simulink library "ddm"  (R2021b)
settings: Solver=VariableStepAuto  StartTime=0.0  StopTime=10.0  RelTol=1e-3
undefined symbols (not defined in the file): ADDM_FrTMTqDev_X_Nm, ADDM_RrTMTqDev_X_Nm, ENUM_ADASACCSTA_ERROR, ENUM_ADASACCSTA_OFF, ENUM_ADASACCSTA_STANDBY, ENUM_ALLOWMOV_ALLOWREADY, ENUM_APS, ENUM_BRKSTA_ERROR, ENUM_BRKSTA_OFF, ENUM_BRKSTA_ON, ENUM_BRKSW_INVALID, ENUM_BRKSW_OFF, ENUM_BRKSW_ON, ENUM_CHGPREACTERRSTA_OBCPRE, ENUM_DCDCFAULTSTA_ANYFAULTLV1, ENUM_DCDCFAULTSTA_ANYFAULTLV2, ENUM_DRIVETRAIN_AWD, ENUM_DRIVETRAIN_FWD, ENUM_DRIVETRAIN_RWD, ENUM_EDUDRTSTA_NORMAL, ENUM_EPBERROR_FAILED, ENUM_EPBSTA_APPLIED, ENUM_EPBSTA_RELEASED, ENUM_ESCAPSSta_APSUNAVAILABLE, ENUM_GEARACTUALPOSN_INVALID, ENUM_GEARACTUALPOSN_P, ENUM_HVBATTREADYPRE_READY, ENUM_HWRESETSTA_HWRESETING, ENUM_MCUWARN_LV0, ENUM_MCUWARN_LV1, ENUM_MCUWARN_LV2, ENUM_MCUWARN_LV3, ENUM_MCUWARN_NOERROR, ENUM_OBCFAULTSTA_ANYFAULT, ENUM_PAS_R2F2, ENUM_PDFAULT_BATTPDFAIL, ENUM_PDFAULT_DCDCDISABLE, ENUM_PDFAULT_MCUDISABLE, ENUM_PDFAULT_MCUDISCHRG, ENUM_POWERSTA_OFF, ENUM_POWERSTA_ON, ENUM_POWERSTA_READY, ENUM_POWERSTA_STANDBY, ENUM_PRESSINDI_LOW, ENUM_PUFAULT_BATTUPFAIL, ENUM_PUFAULT_DCDCENABLEFAIL, ENUM_PUFAULT_PRECHRGCHKFAIL, ENUM_PUFAULT_SAFETYCHKFAIL, ENUM_PWRSTASW_OFF, ENUM_PWRSTASW_OFFA, ENUM_PWRSTASW_OFFCHVCHRG, ENUM_PWRSTASW_OFFCLVCHRG, ENUM_PWRSTASW_ON, ENUM_PWRSTASW_ONHVCHRG, ENUM_PWRSTASW_READY, ENUM_PWRSTASW_STANDBY, ENUM_RAPSErrWarnSta_NORMAL, ENUM_RAPSErrWarnSta_RAPSERRLV1, ENUM_SHIFTCOMMAND_P, ENUM_SHIFTERERRSTA_PBUTTONFAILURE ... (+471)
libraries: hcu_lib x540, simulink x3
(part 24 of 26)

== system ddm/DDM/DDM/VMC_DDM/BMS Signal Error /BMS Signal Error  ==
  note: Test Pass Criteria
  note: Test Detection Criteria
  note: Diagnostics and Fault Handling
  note: Release Condiction After Decision
  task_time_s : Inport
  VDDM_C3BMS6LCCFS_flg : Inport  Port=2
  VDDM_C3BMS6RCCFS_flg : Inport  Port=3
  VDDM_C3BMS6CSCFS_flg : Inport  Port=4
  No_CAN3_BUS_OFF : Inport  Port=5
  VPMM_PowerSta_enum : Inport  Port=6
  VINP_BMSWarn1_flg : Inport  Port=7
  VINP_BMSWarn2_flg : Inport  Port=8
  VINP_BMSWarn3_flg : Inport  Port=9
  DTC_clear_request : Inport  Port=10
  VINP_BMSWarn4_flg : Inport  Port=11
  VINP_BMSWarn5_flg : Inport  Port=12
  VINP_BMSWarn6_flg : Inport  Port=13
  VINP_BMSWarn7_flg : Inport  Port=14
  VINP_BMSWarn8_flg : Inport  Port=15
  Constant : Constant  Value=ENUM_POWERSTA_OFF
  Constant1 : Constant  Value=ENUM_POWERSTA_OFF
  Constant10 : Constant  Value=ZERO_INT
  Constant12 : Constant  Value=KDDM_BMSSigErrDTC_cnt
  Constant16 : Constant  Value=ENUM_POWERSTA_OFF
  Constant17 : Constant  Value=ENUM_POWERSTA_STANDBY
  Constant18 : Constant  Value=TRUE
  Constant19 : Constant  Value=FALSE
  Constant2 : Constant  Value=FALSE
  Constant3 : Constant  Value=FALSE
  Constant4 : Constant  Value=KDDM_BMSSigErrDetTO_s
  Constant5 : Constant  Value=TRUE
  Constant6 : Constant  Value=KDDM_BMSSigErrPassTO_s
  Constant7 : Constant  Value=KDDM_BMSSigErrDTC_cnt
  Constant8 : Constant  Value=KDDM_VMCDiagnosisOffSW_flg
  Constant9 : Constant  Value=KDDM_BMSSigErrPassTO_s
  DTC_Couter1 : hcu_lib/Basic_Blocks/DTC_Couter
  DTC_Info : hcu_lib/Basic_Blocks/DTC_Info
  Equal : RelationalOperator  Operator=~=  OutDataTypeStr=boolean  RndMeth=Simplest
  Equal1 : RelationalOperator  Operator=~=  OutDataTypeStr=boolean  RndMeth=Simplest
  Equal2 : RelationalOperator  Operator===  OutDataTypeStr=boolean  RndMeth=Simplest
  Equal3 : RelationalOperator  OutDataTypeStr=boolean  RndMeth=Simplest
  Equal4 : RelationalOperator  Operator===  OutDataTypeStr=boolean  RndMeth=Simplest
  Logical Operator1 : Logic  Operator=OR  Inputs=4  AllPortsSameDT=off  OutDataTypeStr=boolean
  Logical Operator10 : Logic  AllPortsSameDT=off  OutDataTypeStr=boolean
  Logical Operator16 : Logic  Operator=OR  Inputs=8  AllPortsSameDT=off  OutDataTypeStr=boolean
  Logical Operator{6,17..18,20..22,24} (7 alike) : Logic  Operator=NOT  AllPortsSameDT=off  OutDataTypeStr=boolean
  Logical Operator2 : Logic  Inputs=5  AllPortsSameDT=off  OutDataTypeStr=boolean
  Logical Operator23 : Logic  Inputs=5  AllPortsSameDT=off  OutDataTypeStr=boolean
  Logical Operator4 : Logic  Operator=OR  Inputs=8  AllPortsSameDT=off  OutDataTypeStr=boolean
  Relational Operator : RelationalOperator  Operator=>  OutDataTypeStr=boolean  RndMeth=Simplest
  Switch{2..3,5..6} (4 alike) : Switch  Criteria=u2 ~= 0
  Terminator : Terminator
  Test Detection Criteria : hcu_lib/Basic_Blocks/Test Detection Criteria
  Timer1 : hcu_lib/Basic_Blocks/Timer
  Unit Delay1 : UnitDelay  SampleTime=-1  HasFrameUpgradeWarning=on
  VDDM_BMSSigErrCFS_flg : Outport
  VDDM_BMSSigErrDetDTC_raw32 : Outport  Port=2
  wires:
  [VDDM_BMSSigErrPass_flg] -> Logical Operator1/1
  Switch6/1 -> [VDDM_BMSSigErrCFSRls_flg]  "VDDM_BMSSigErrCFSRls_flg"
  Equal4/1 -> Logical Operator10/2
  Constant17/1 -> Equal4/2
  DTC_Couter1/2 -> Relational Operator/1  "VDDM_BMSSigErrDTC_cnt"
  Unit Delay1/1 -> Equal2/1
  Logical Operator10/1 -> Logical Operator1/2
  Logical Operator1/1 -> Switch6/2
  Constant16/1 -> Equal2/2
  [VPMM_PowerSta_enum] -> Equal4/1
  Constant18/1 -> Switch6/1
  [VDDM_BMSSigErrCFSRls_flg] -> DTC_Couter1/2
  Constant12/1 -> DTC_Couter1/3
  [DTC_clear_request] -> Logical Operator1/3
  [VDDM_BMSSigErrDet_flg] -> DTC_Couter1/1
  Relational Operator/1 -> Terminator/1  "VDDM_BMSSigErrDFS_flg"
  DTC_Couter1/1 -> [VDDM_BMSSigErrCFS_flg]  "VDDM_BMSSigErrCFS_flg"
  Constant10/1 -> Relational Operator/2
  Constant8/1 -> Logical Operator1/4
  [VPMM_PowerSta_enum] -> Unit Delay1/1
  Constant19/1 -> Switch6/3
  Equal2/1 -> Logical Operator10/1
  Equal3/1 -> [VDDM_BMSSigErrPass_flg]  "VDDM_BMSSigErrPass_flg"
  [task_time_s] -> Timer1/3
  Constant4/1 -> Test Detection Criteria/4
  [VINP_BMSWarn8_flg] -> Logical Operator4/8
  [VINP_BMSWarn7_flg] -> Logical Operator4/7
  [VINP_BMSWarn6_flg] -> Logical Operator4/6
  [VINP_BMSWarn5_flg] -> Logical Operator4/5
  [VINP_BMSWarn8_flg] -> Logical Operator16/8
  [VINP_BMSWarn7_flg] -> Logical Operator16/7
  [VINP_BMSWarn6_flg] -> Logical Operator16/6
  [VINP_BMSWarn5_flg] -> Logical Operator16/5
  [VINP_BMSWarn4_flg] -> Logical Operator16/4
  VINP_BMSWarn8_flg/1 -> [VINP_BMSWarn8_flg]
  VINP_BMSWarn7_flg/1 -> [VINP_BMSWarn7_flg]
  VINP_BMSWarn6_flg/1 -> [VINP_BMSWarn6_flg]
  VINP_BMSWarn5_flg/1 -> [VINP_BMSWarn5_flg]
  VINP_BMSWarn4_flg/1 -> [VINP_BMSWarn4_flg]
  DTC_Info/1 -> VDDM_BMSSigErrDetDTC_raw32/1  "VDDM_BMSSigErrDetDTC_raw32"
  [DTC_clear_request] -> DTC_Info/4
  [VDDM_BMSSigErrCFS_flg] -> DTC_Info/3
  [VDDM_BMSSigErrPass_flg] -> DTC_Info/2
  [VDDM_BMSSigErrDet_flg] -> DTC_Info/1
  Switch5/1 -> Test Detection Criteria/1
  [VDDM_BMSSigErrCFSRls_flg] -> Switch5/2
  Constant3/1 -> Switch5/1
  Constant9/1 -> Timer1/4
  Test Detection Criteria/1 -> [VDDM_BMSSigErrDet_flg]  "VDDM_BMSSigErrDet_flg"
  Constant7/1 -> Test Detection Criteria/3
  [task_time_s] -> Test Detection Criteria/2
  task_time_s/1 -> [task_time_s]  "task_time_s"
  Switch3/1 -> Logical Operator6/1, Timer1/2
  Constant1/1 -> Equal1/2
  [No_CAN3_BUS_OFF] -> Logical Operator23/1
  [VDDM_C3BMS6CSCFS_flg] -> Logical Operator24/1
  Logical Operator21/1 -> Logical Operator23/2
  Logical Operator24/1 -> Logical Operator23/4
  [VDDM_C3BMS6RCCFS_flg] -> Logical Operator22/1
  Equal1/1 -> Logical Operator23/5
  Constant5/1 -> Switch3/3
  Logical Operator23/1 -> Switch3/2
  [VPMM_PowerSta_enum] -> Equal1/1
  Logical Operator4/1 -> Switch3/1
  [VDDM_C3BMS6LCCFS_flg] -> Logical Operator21/1
  Logical Operator22/1 -> Logical Operator23/3
  Logical Operator20/1 -> Logical Operator2/4
  Logical Operator18/1 -> Logical Operator2/3
  Logical Operator17/1 -> Logical Operator2/2
  [VINP_BMSWarn3_flg] -> Logical Operator16/3
  [VINP_BMSWarn2_flg] -> Logical Operator16/2
  [VINP_BMSWarn1_flg] -> Logical Operator16/1
  Logical Operator16/1 -> Switch2/1
  [VDDM_C3BMS6CSCFS_flg] -> Logical Operator20/1
  [VDDM_C3BMS6RCCFS_flg] -> Logical Operator18/1
  [VDDM_C3BMS6LCCFS_flg] -> Logical Operator17/1
  Equal/1 -> Logical Operator2/5
  VINP_BMSWarn1_flg/1 -> [VINP_BMSWarn1_flg]
  No_CAN3_BUS_OFF/1 -> [No_CAN3_BUS_OFF]
  VDDM_C3BMS6CSCFS_flg/1 -> [VDDM_C3BMS6CSCFS_flg]
  VINP_BMSWarn2_flg/1 -> [VINP_BMSWarn2_flg]
  VPMM_PowerSta_enum/1 -> [VPMM_PowerSta_enum]
  VDDM_C3BMS6RCCFS_flg/1 -> [VDDM_C3BMS6RCCFS_flg]
  DTC_clear_request/1 -> [DTC_clear_request]
  VDDM_C3BMS6LCCFS_flg/1 -> [VDDM_C3BMS6LCCFS_flg]
  VINP_BMSWarn3_flg/1 -> [VINP_BMSWarn3_flg]
  Timer1/1 -> Equal3/1
  [VPMM_PowerSta_enum] -> Equal/1
  Constant2/1 -> Switch2/3
  Constant/1 -> Equal/2
  Logical Operator6/1 -> Timer1/1
  Logical Operator2/1 -> Switch2/2
  [No_CAN3_BUS_OFF] -> Logical Operator2/1
  Constant6/1 -> Equal3/2
  [VDDM_BMSSigErrCFS_flg] -> VDDM_BMSSigErrCFS_flg/1
  Switch2/1 -> Switch5/3
  [VINP_BMSWarn1_flg] -> Logical Operator4/1
  [VINP_BMSWarn2_flg] -> Logical Operator4/2
  [VINP_BMSWarn3_flg] -> Logical Operator4/3
  [VINP_BMSWarn4_flg] -> Logical Operator4/4

== system ddm/DDM/DDM/VMC_DDM/CCU Signal Error/CCU Signal Error  ==
  note: Test Pass Criteria
  note: Test Detection Criteria
  note: Release Condiction After Decision
  note: Diagnostics and Fault Handling
  task_time_s : Inport
  VDDM_C3CCU2LCCFS_flg : Inport  Port=2
  VDDM_C3CCU2RCCFS_flg : Inport  Port=3
  VDDM_C3CCU2CSCFS_flg : Inport  Port=4
  No_CAN3_BUS_OFF : Inport  Port=5
  VPMM_PowerSta_enum : Inport  Port=6
  VINP_DCDCFaultSta_enum : Inport  Port=7
  DTC_clear_request : Inport  Port=8
  Constant : Constant  Value=ENUM_POWERSTA_OFF
  Constant1 : Constant  Value=ENUM_POWERSTA_OFF
  Constant10 : Constant  Value=FALSE
  Constant12 : Constant  Value=KDDM_CCUSigErrDTC_cnt
  Constant2 : Constant  Value=FALSE
  Constant21 : Constant  Value=ZERO_INT
  Constant3 : Constant  Value=ENUM_DCDCFAULTSTA_ANYFAULTLV1
  Constant30 : Constant  Value=ENUM_POWERSTA_OFF
  Constant31 : Constant  Value=ENUM_POWERSTA_STANDBY
  Constant32 : Constant  Value=TRUE
  Constant37 : Constant  Value=FALSE
  Constant38 : Constant  Value=KDDM_VMCDiagnosisOffSW_flg
  Constant4 : Constant  Value=KDDM_CCUSigErrDetTO_s
  Constant5 : Constant  Value=TRUE
  Constant6 : Constant  Value=KDDM_CCUSigErrPassTO_s
  Constant7 : Constant  Value=KDDM_CCUSigErrDTC_cnt
  Constant8 : Constant  Value=ENUM_DCDCFAULTSTA_ANYFAULTLV1
  Constant9 : Constant  Value=KDDM_CCUSigErrPassTO_s
  DTC_Couter1 : hcu_lib/Basic_Blocks/DTC_Couter
  DTC_Info : hcu_lib/Basic_Blocks/DTC_Info
  Equal : RelationalOperator  Operator=~=  OutDataTypeStr=boolean  RndMeth=Simplest
  Equal1 : RelationalOperator  Operator=~=  OutDataTypeStr=boolean  RndMeth=Simplest
  Equal17 : RelationalOperator  Operator===  OutDataTypeStr=boolean  RndMeth=Simplest
  Equal18 : RelationalOperator  Operator===  OutDataTypeStr=boolean  RndMeth=Simplest
  Equal2 : RelationalOperator  OutDataTypeStr=boolean  RndMeth=Simplest
  Equal3 : RelationalOperator  OutDataTypeStr=boolean  RndMeth=Simplest
  Equal4 : RelationalOperator  OutDataTypeStr=boolean  RndMeth=Simplest
  Logical Operator10 : Logic  AllPortsSameDT=off  OutDataTypeStr=boolean
  Logical Operator{6,17..18,20..22,24} (7 alike) : Logic  Operator=NOT  AllPortsSameDT=off  OutDataTypeStr=boolean
  Logical Operator2 : Logic  Inputs=5  AllPortsSameDT=off  OutDataTypeStr=boolean
  Logical Operator23 : Logic  Inputs=5  AllPortsSameDT=off  OutDataTypeStr=boolean
  Logical Operator4 : Logic  Operator=OR  Inputs=4  AllPortsSameDT=off  OutDataTypeStr=boolean
  Relational Operator : RelationalOperator  Operator=>  OutDataTypeStr=boolean  RndMeth=Simplest
  Switch{2..3,5..6} (4 alike) : Switch  Criteria=u2 ~= 0
  Terminator : Terminator
  Test Detection Criteria : hcu_lib/Basic_Blocks/Test Detection Criteria
  Timer1 : hcu_lib/Basic_Blocks/Timer
  Unit Delay1 : UnitDelay  SampleTime=-1  HasFrameUpgradeWarning=on
  VDDM_CCUSigErrCFS_flg : Outport
  VDDM_CCUSigErrDetDTC_raw32 : Outport  Port=2
  wires:
  Constant31/1 -> Equal18/2
  Switch6/1 -> [VDDM_CCUSigErrCFSRls_flg]  "VDDM_CCUSigErrCFSRls_flg"
  Constant21/1 -> Relational Operator/2
  Constant30/1 -> Equal17/2
  Equal18/1 -> Logical Operator10/2
  [VDDM_CCUSigErrCFSRls_flg] -> DTC_Couter1/2
  [VDDM_CCUSigErrPass_flg] -> Logical Operator4/1
  Logical Operator10/1 -> Logical Operator4/2
  DTC_Couter1/2 -> Relational Operator/1  "VDDM_CCUSigErrDTC_cnt"
  [DTC_clear_request] -> Logical Operator4/3
  Constant32/1 -> Switch6/1
  Constant38/1 -> Logical Operator4/4
  [VPMM_PowerSta_enum] -> Unit Delay1/1
  Unit Delay1/1 -> Equal17/1
  [VPMM_PowerSta_enum] -> Equal18/1
  Logical Operator4/1 -> Switch6/2
  Constant37/1 -> Switch6/3
  Equal17/1 -> Logical Operator10/1
  DTC_Couter1/1 -> [VDDM_CCUSigErrCFS_flg]  "VDDM_CCUSigErrCFS_flg"
  Constant12/1 -> DTC_Couter1/3
  [VDDM_CCUSigErrDet_flg] -> DTC_Couter1/1
  Relational Operator/1 -> Terminator/1  "VDDM_CCUSigErrDFS_flg"
  DTC_Info/1 -> VDDM_CCUSigErrDetDTC_raw32/1  "VDDM_CCUSigErrDetDTC_raw32"
  [DTC_clear_request] -> DTC_Info/4
  [VDDM_CCUSigErrCFS_flg] -> DTC_Info/3
  [VDDM_CCUSigErrPass_flg] -> DTC_Info/2
  [VDDM_CCUSigErrDet_flg] -> DTC_Info/1
  Switch5/1 -> Test Detection Criteria/1
  Constant10/1 -> Switch5/1
  [VDDM_CCUSigErrCFSRls_flg] -> Switch5/2
  Equal4/1 -> Switch3/1
  Constant8/1 -> Equal4/2
  [VINP_DCDCFaultSta_enum] -> Equal4/1
  Equal2/1 -> Switch2/1
  Constant3/1 -> Equal2/2
  Constant9/1 -> Timer1/4
  [task_time_s] -> Timer1/3
  Test Detection Criteria/1 -> [VDDM_CCUSigErrDet_flg]  "VDDM_CCUSigErrDet_flg"
  Constant7/1 -> Test Detection Criteria/3
  Constant4/1 -> Test Detection Criteria/4
  [task_time_s] -> Test Detection Criteria/2
  task_time_s/1 -> [task_time_s]  "task_time_s"
  Switch3/1 -> Logical Operator6/1, Timer1/2
  Constant1/1 -> Equal1/2
  [No_CAN3_BUS_OFF] -> Logical Operator23/1
  [VDDM_C3CCU2CSCFS_flg] -> Logical Operator24/1
  Logical Operator21/1 -> Logical Operator23/2
  Logical Operator24/1 -> Logical Operator23/4
  [VDDM_C3CCU2RCCFS_flg] -> Logical Operator22/1
  Equal1/1 -> Logical Operator23/5
  Constant5/1 -> Switch3/3
  Logical Operator23/1 -> Switch3/2
  [VPMM_PowerSta_enum] -> Equal1/1
  [VDDM_C3CCU2LCCFS_flg] -> Logical Operator21/1
  Logical Operator22/1 -> Logical Operator23/3
  Logical Operator20/1 -> Logical Operator2/4
  Logical Operator18/1 -> Logical Operator2/3
  Logical Operator17/1 -> Logical Operator2/2
  [VINP_DCDCFaultSta_enum] -> Equal2/1
  [VDDM_C3CCU2CSCFS_flg] -> Logical Operator20/1
  [VDDM_C3CCU2RCCFS_flg] -> Logical Operator18/1
  [VDDM_C3CCU2LCCFS_flg] -> Logical Operator17/1
  Equal/1 -> Logical Operator2/5
  VINP_DCDCFaultSta_enum/1 -> [VINP_DCDCFaultSta_enum]
  No_CAN3_BUS_OFF/1 -> [No_CAN3_BUS_OFF]
  VDDM_C3CCU2CSCFS_flg/1 -> [VDDM_C3CCU2CSCFS_flg]
  VPMM_PowerSta_enum/1 -> [VPMM_PowerSta_enum]
  VDDM_C3CCU2RCCFS_flg/1 -> [VDDM_C3CCU2RCCFS_flg]
  DTC_clear_request/1 -> [DTC_clear_request]
  VDDM_C3CCU2LCCFS_flg/1 -> [VDDM_C3CCU2LCCFS_flg]
  Timer1/1 -> Equal3/1
  [VPMM_PowerSta_enum] -> Equal/1
  Constant2/1 -> Switch2/3
  Constant/1 -> Equal/2
  Logical Operator6/1 -> Timer1/1
  Logical Operator2/1 -> Switch2/2
  [No_CAN3_BUS_OFF] -> Logical Operator2/1
  Constant6/1 -> Equal3/2
  [VDDM_CCUSigErrCFS_flg] -> VDDM_CCUSigErrCFS_flg/1
  Equal3/1 -> [VDDM_CCUSigErrPass_flg]  "VDDM_CCUSigErrPass_flg"
  Switch2/1 -> Switch5/3

== system ddm/DDM/DDM/VMC_DDM/ESC Signal Error/ESC Signal Error  ==
  note: Test Detection Criteria
  note: Test Pass Criteria
  note: Release Condiction After Decision
  note: Diagnostics and Fault Handling
  task_time_s : Inport
  No_CAN1_BUS_OFF : Inport  Port=2
  VPMM_PowerSta_enum : Inport  Port=3
  DTC_clear_request : Inport  Port=4
  VINP_ABSFailed_flg : Inport  Port=5
  VINP_TCSFailed_flg : Inport  Port=6
  VINP_ESCFailed_flg : Inport  Port=7
  VINP_HSAFailed_flg : Inport  Port=8
  VINP_AVHFailed_flg : Inport  Port=9
  VINP_MCPressureV_flg : Inport  Port=10
  VINP_BrkSwV_flg : Inport  Port=11
  VINP_BrkPedalPosSta_flg : Inport  Port=12
  VINP_LongAccelV_flg : Inport  Port=13
  VINP_LatAccelV_flg : Inport  Port=14
  VINP_YawRateV_flg : Inport  Port=15
  VINP_LRRawWhlSpeedV_flg : Inport  Port=16
  VINP_RRRawWhlSpeedV_flg : Inport  Port=17
  VINP_LFRawWhlSpeedV_flg : Inport  Port=18
  VINP_RFRawWhlSpeedV_flg : Inport  Port=19
  VINP_VehSpeed_kph : Inport  Port=20
  VINP_FrntAxlTrqReqDrv_Nm : Inport  Port=21
  VINP_RearAxlTrqReqDrv_Nm : Inport  Port=22
  VDDM_ESC1Err_flg : Inport  Port=23
  VDDM_ESC5Err_flg : Inport  Port=24
  VINP_GRADE_Deg : Inport  Port=25
  VINP_FrntAxlTrqReqBrk_Nm : Inport  Port=26
  VINP_RearAxlTrqReqBrk_Nm : Inport  Port=27
  VINP_ESCAPSSta_enum : Inport  Port=28
  AND : Logic  AllPortsSameDT=off  OutDataTypeStr=boolean
  AND1 : Logic  AllPortsSameDT=off  OutDataTypeStr=boolean
  Constant : Constant  Value=ENUM_POWERSTA_OFF
  Constant1 : Constant  Value=ENUM_POWERSTA_OFF
  Constant10 : Constant  Value=ZERO_INT
  Constant11 : Constant  Value=KDDM_VMCDiagnosisOffSW_flg
  Constant12 : Constant  Value=ENUM_POWERSTA_OFF
  Constant13 : Constant  Value=ENUM_POWERSTA_STANDBY
  Constant14 : Constant  Value=TRUE
  Constant15 : Constant  Value=FALSE
  Constant16 : Constant  Value=FALSE
  Constant17 : Constant  Value=45  OutDataTypeStr=single
  Constant18 : Constant  Value=ZERO_FLOAT  OutDataTypeStr=single
  Constant19 : Constant  Value=ZERO_FLOAT  OutDataTypeStr=single
  Constant2 : Constant  Value=FALSE
  Constant20 : Constant  Value=TRUE
  Constant21 : Constant  Value=ENUM_ESCAPSSta_APSUNAVAILABLE  OutDataTypeStr=single
  Constant34 : Constant  Value=KDDM_ESCSigErrDTC_cnt
  Constant4 : Constant  Value=KDDM_ESCSigErrDetTO_s
  Constant5 : Constant  Value=5300  OutDataTypeStr=single
  Constant6 : Constant  Value=KDDM_ESCSigErrPassTO_s
  Constant66 : Constant  Value=255  OutDataTypeStr=single
  Constant7 : Constant  Value=KDDM_ESCSigErrDTC_cnt
  Constant8 : Constant  Value=5300  OutDataTypeStr=single
  Constant9 : Constant  Value=KDDM_ESCSigErrPassTO_s
  DTC_Couter : hcu_lib/Basic_Blocks/DTC_Couter
  DTC_Info : hcu_lib/Basic_Blocks/DTC_Info
  Data Type Conversion{,1..3} (4 alike) : DataTypeConversion  OutDataTypeStr=single
  Equal : RelationalOperator  Operator=~=  OutDataTypeStr=boolean  RndMeth=Simplest
  Equal1 : RelationalOperator  Operator=~=  OutDataTypeStr=boolean  RndMeth=Simplest
  Equal{2,4..5,54} (4 alike) : RelationalOperator  Operator=>  OutDataTypeStr=boolean  RndMeth=Simplest
  Equal3 : RelationalOperator  OutDataTypeStr=boolean  RndMeth=Simplest
  Equal6 : RelationalOperator  Operator===  OutDataTypeStr=boolean  RndMeth=Simplest
  Equal7 : RelationalOperator  Operator===  OutDataTypeStr=boolean  RndMeth=Simplest
  Logical Operator1 : Logic  AllPortsSameDT=off  OutDataTypeStr=boolean
  Logical Operator2 : Logic  AllPortsSameDT=off  OutDataTypeStr=boolean
  Logical Operator6 : Logic  Operator=NOT  AllPortsSameDT=off  OutDataTypeStr=boolean
  Logical Operator8 : Logic  Operator=OR  Inputs=4  AllPortsSameDT=off  OutDataTypeStr=boolean
  Logical Operator9 : Logic  AllPortsSameDT=off  OutDataTypeStr=boolean
  NOT1 : Logic  Operator=NOT  AllPortsSameDT=off  OutDataTypeStr=boolean
  NOT2 : Logic  Operator=NOT  AllPortsSameDT=off  OutDataTypeStr=boolean
  NOT9 : Logic  Operator=NOT  AllPortsSameDT=off  OutDataTypeStr=boolean
  OR : Logic  Operator=OR  Inputs=13  AllPortsSameDT=off  OutDataTypeStr=boolean
  OR1 : Logic  Operator=OR  Inputs=9  AllPortsSameDT=off  OutDataTypeStr=boolean
  OR2 : Logic  Operator=OR  AllPortsSameDT=off  OutDataTypeStr=boolean
  OR3 : Logic  Operator=OR  AllPortsSameDT=off  OutDataTypeStr=boolean
  Relational Operator : RelationalOperator  Operator=>  OutDataTypeStr=boolean  RndMeth=Simplest
  Relational Operator1 : RelationalOperator  Operator=>  OutDataTypeStr=boolean  RndMeth=Simplest
  Relational Operator2 : RelationalOperator  Operator=>  OutDataTypeStr=boolean  RndMeth=Simplest
  Relational Operator5 : RelationalOperator  Operator===  OutDataTypeStr=boolean  RndMeth=Simplest
  Switch{1..2,4..5} (4 alike) : Switch  Criteria=u2 ~= 0
  Terminator : Terminator
  Test Detection Criteria : hcu_lib/Basic_Blocks/Test Detection Criteria
  Timer1 : hcu_lib/Basic_Blocks/Timer
  Unit Delay2 : UnitDelay  SampleTime=-1  HasFrameUpgradeWarning=on
  VDDM_ESCSigErrCFS_flg : Outport
  VDDM_ESCSigErrDetDTC_raw32 : Outport  Port=2
  VDDM_ESC1SigErr_flg : Outport  Port=3
  VDDM_ESC5SigErr_flg : Outport  Port=4
  wires:
  [DTC_clear_request] -> DTC_Info/4
  [VDDM_ESCSigErrCFS_flg] -> DTC_Info/3
  [VDDM_ESCSigErrPass_flg] -> DTC_Info/2
  [VDDM_ESCSigErrDet_flg] -> DTC_Info/1
  DTC_Info/1 -> [VDDM_ESCSigErrDetDTC_raw32]  "VDDM_ESCSigErrDetDTC_raw32"
  Switch5/1 -> Test Detection Criteria/1
  [VDDM_ESCSigErrCFSRls_flg] -> Switch5/2
  Constant16/1 -> Switch5/1
  [VDDM_ESC5SigErr_flg] -> VDDM_ESC5SigErr_flg/1
  [VDDM_ESC1SigErr_flg] -> VDDM_ESC1SigErr_flg/1
  VINP_RFRawWhlSpeedV_flg/1 -> [VINP_RFRawWhlSpeedV_flg]
  VINP_LFRawWhlSpeedV_flg/1 -> [VINP_LFRawWhlSpeedV_flg]
  VINP_RRRawWhlSpeedV_flg/1 -> [VINP_RRRawWhlSpeedV_flg]
  VINP_LRRawWhlSpeedV_flg/1 -> [VINP_LRRawWhlSpeedV_flg]
  Constant11/1 -> Logical Operator8/4
  [VPMM_PowerSta_enum] -> Equal1/1
  Constant1/1 -> Equal1/2
  Logical Operator1/1 -> Switch1/2
  [VDDM_ESC5SigErr_flg] -> OR3/2
  [VDDM_ESC1SigErr_flg] -> OR3/1
  [No_CAN1_BUS_OFF] -> Logical Operator1/1
  Constant20/1 -> Switch1/3
  OR3/1 -> Switch1/1
  Equal1/1 -> Logical Operator1/2
  [VDDM_ESC5SigErr_flg] -> OR2/2
  AND1/1 -> [VDDM_ESC5SigErr_flg]  "VDDM_ESC5SigErr_flg"
  NOT2/1 -> AND1/2
  AND/1 -> [VDDM_ESC1SigErr_flg]  "VDDM_ESC1SigErr_flg"
  VINP_LatAccelV_flg/1 -> [VINP_LatAccelV_flg]
  VINP_YawRateV_flg/1 -> [VINP_YawRateV_flg]
  VINP_LongAccelV_flg/1 -> [VINP_LongAccelV_flg]
  VINP_BrkPedalPosSta_flg/1 -> [VINP_BrkPedalPosSta_flg]
  VINP_BrkSwV_flg/1 -> [VINP_BrkSwV_flg]
  VINP_ABSFailed_flg/1 -> [VINP_ABSFailed_flg]
  VINP_TCSFailed_flg/1 -> [VINP_TCSFailed_flg]
  VINP_ESCFailed_flg/1 -> [VINP_ESCFailed_flg]
  VINP_HSAFailed_flg/1 -> [VINP_HSAFailed_flg]
  VINP_MCPressureV_flg/1 -> [VINP_MCPressureV_flg]
  VINP_AVHFailed_flg/1 -> [VINP_AVHFailed_flg]
  Equal3/1 -> [VDDM_ESCSigErrPass_flg]  "VDDM_ESCSigErrPass_flg"
  [VDDM_ESCSigErrCFS_flg] -> VDDM_ESCSigErrCFS_flg/1
  Constant15/1 -> Switch4/3
  Equal6/1 -> Logical Operator9/1
  Equal7/1 -> Logical Operator9/2
  Constant6/1 -> Equal3/2
  [VPMM_PowerSta_enum] -> Unit Delay2/1
  Logical Operator9/1 -> Logical Operator8/2
  Switch4/1 -> [VDDM_ESCSigErrCFSRls_flg]  "VDDM_ESCSigErrCFSRls_flg"
  [No_CAN1_BUS_OFF] -> Logical Operator2/1
  [VDDM_ESCSigErrPass_flg] -> Logical Operator8/1
  [DTC_clear_request] -> Logical Operator8/3
  Logical Operator2/1 -> Switch2/2
  Logical Operator6/1 -> Timer1/1
  Constant13/1 -> Equal7/2
  Constant/1 -> Equal/2
  Unit Delay2/1 -> Equal6/1
  Constant12/1 -> Equal6/2
  Constant2/1 -> Switch2/3
  Constant14/1 -> Switch4/1
  [VPMM_PowerSta_enum] -> Equal7/1
  Logical Operator8/1 -> Switch4/2
  [VPMM_PowerSta_enum] -> Equal/1
  Timer1/1 -> Equal3/1
  DTC_clear_request/1 -> [DTC_clear_request]
  VPMM_PowerSta_enum/1 -> [VPMM_PowerSta_enum]
  No_CAN1_BUS_OFF/1 -> [No_CAN1_BUS_OFF]
  Equal/1 -> Logical Operator2/2
  Switch1/1 -> Logical Operator6/1, Timer1/2
  task_time_s/1 -> [task_time_s]  "task_time_s"
  [task_time_s] -> Test Detection Criteria/2
  Constant4/1 -> Test Detection Criteria/4
  Constant7/1 -> Test Detection Criteria/3
  Test Detection Criteria/1 -> [VDDM_ESCSigErrDet_flg]  "VDDM_ESCSigErrDet_flg"
  [task_time_s] -> Timer1/3
  Constant9/1 -> Timer1/4
  DTC_Couter/2 -> Relational Operator/1  "VDDM_ESCSigErrDTC_cnt"
  Constant34/1 -> DTC_Couter/3
  [VDDM_ESCSigErrCFSRls_flg] -> DTC_Couter/2
  [VDDM_ESCSigErrDet_flg] -> DTC_Couter/1
  Relational Operator/1 -> Terminator/1  "VDDM_ESCSigErrDFS_flg"
  DTC_Couter/1 -> [VDDM_ESCSigErrCFS_flg]  "VDDM_ESCSigErrCFS_flg"
  OR2/1 -> Switch2/1
  Switch2/1 -> Switch5/3
  Constant10/1 -> Relational Operator/2
  [VDDM_ESCSigErrDetDTC_raw32] -> VDDM_ESCSigErrDetDTC_raw32/1
  [VDDM_ESC1SigErr_flg] -> OR2/1
  [VINP_AVHFailed_flg] -> OR/9
  Data Type Conversion3/1 -> Equal54/2
  [VINP_LFRawWhlSpeedV_flg] -> OR/11
  [VINP_ESCFailed_flg] -> OR/7
  Constant66/1 -> Data Type Conversion3/1
  [VINP_RRRawWhlSpeedV_flg] -> OR/12
  Constant8/1 -> Data Type Conversion1/1
  [VINP_LRRawWhlSpeedV_flg] -> OR/13
  [VINP_GRADE_Deg] -> Equal5/1
  [VINP_TCSFailed_flg] -> OR/6
  Equal2/1 -> OR/2
  Data Type Conversion2/1 -> Equal2/2
  [VINP_ABSFailed_flg] -> OR/5
  Equal5/1 -> OR/4
  Data Type Conversion/1 -> Equal5/2
  [VINP_FrntAxlTrqReqDrv_Nm] -> Equal2/1
  Equal54/1 -> OR/1
  Constant17/1 -> Data Type Conversion/1
  Equal4/1 -> OR/3
  [VINP_RFRawWhlSpeedV_flg] -> OR/10
  [VINP_VehSpeed_kph] -> Equal54/1
  [VINP_RearAxlTrqReqDrv_Nm] -> Equal4/1
  [VINP_HSAFailed_flg] -> OR/8
  Data Type Conversion1/1 -> Equal4/2
  Constant5/1 -> Data Type Conversion2/1
  OR/1 -> AND/1
  [VINP_ESCAPSSta_enum] -> Relational Operator5/1
  Relational Operator5/1 -> OR1/9
  Relational Operator1/1 -> OR1/7
  [VINP_FrntAxlTrqReqBrk_Nm] -> Relational Operator1/1
  Constant21/1 -> Relational Operator5/2
  [VINP_RearAxlTrqReqBrk_Nm] -> Relational Operator2/1
  Relational Operator2/1 -> OR1/8
  [VINP_LatAccelV_flg] -> OR1/4
  NOT9/1 -> OR1/6
  [VINP_MCPressureV_flg] -> OR1/1
  Constant19/1 -> Relational Operator1/2
  [VINP_LongAccelV_flg] -> OR1/3
  [VINP_BrkSwV_flg] -> OR1/2
  Constant18/1 -> Relational Operator2/2
  [VINP_YawRateV_flg] -> OR1/5
  [VINP_BrkPedalPosSta_flg] -> NOT9/1
  OR1/1 -> AND1/1
  VDDM_ESC5Err_flg/1 -> [VDDM_ESC5Err_flg]
  VINP_ESCAPSSta_enum/1 -> [VINP_ESCAPSSta_enum]
  VDDM_ESC1Err_flg/1 -> [VDDM_ESC1Err_flg]
  VINP_FrntAxlTrqReqDrv_Nm/1 -> [VINP_FrntAxlTrqReqDrv_Nm]
  VINP_RearAxlTrqReqDrv_Nm/1 -> [VINP_RearAxlTrqReqDrv_Nm]
  VINP_FrntAxlTrqReqBrk_Nm/1 -> [VINP_FrntAxlTrqReqBrk_Nm]
  VINP_GRADE_Deg/1 -> [VINP_GRADE_Deg]
  VINP_VehSpeed_kph/1 -> [VINP_VehSpeed_kph]
  VINP_RearAxlTrqReqBrk_Nm/1 -> [VINP_RearAxlTrqReqBrk_Nm]
  NOT1/1 -> AND/2
  [VDDM_ESC1Err_flg] -> NOT1/1
  [VDDM_ESC5Err_flg] -> NOT2/1

== system ddm/DDM/DDM/VMC_DDM/Enabled Subsystem/EPS1 Checksum Error ==
  note: Test Pass Criteria
  note: Test Detection Criteria
  note: Diagnostics and Fault Handling
  note: Release Condiction After Decision
  task_time_s : Inport
  VDDM_EPSCSErr_flg : Inport  Port=2
  No_CAN1_BUS_OFF : Inport  Port=3
  VDDM_EPS1NoComCFS_flg : Inport  Port=4
  VPMM_PowerSta_enum : Inport  Port=5
  DTC_clear_request : Inport  Port=6
  VTQD_GearActualPosn_enum : Inport  Port=7
  Constant : Constant  Value=ENUM_POWERSTA_OFF
  Constant1 : Constant  Value=ENUM_POWERSTA_OFF
  Constant10 : Constant  Value=FALSE
  Constant11 : Constant  Value=ZERO_INT
  Constant12 : Constant  Value=KDDM_EPS1CSErrDTC_cnt
  Constant13 : Constant  Value=KDDM_VMCDiagnosisOffSW_flg
  Constant2 : Constant  Value=FALSE
  Constant3 : Constant  Value=TRUE
  Constant4 : Constant  Value=ENUM_GEARACTUALPOSN_P
  Constant40 : Constant  Value=KDDM_EPS1CSErrDTC_cnt
  Constant41 : Constant  Value=KDDM_EPS1CSErrDetTO_s
  Constant49 : Constant  Value=ENUM_POWERSTA_OFF
  Constant52 : Constant  Value=ENUM_POWERSTA_STANDBY
  Constant6 : Constant  Value=KDDM_EPS1CSErrPassTO_s
  Constant9 : Constant  Value=KDDM_EPS1CSErrPassTO_s
  DTC_Couter2 : hcu_lib/Basic_Blocks/DTC_Couter
  DTC_Info : hcu_lib/Basic_Blocks/DTC_Info
  Equal : RelationalOperator  Operator=~=  OutDataTypeStr=boolean  RndMeth=Simplest
  Equal1 : RelationalOperator  Operator=~=  OutDataTypeStr=boolean  RndMeth=Simplest
  Equal2 : RelationalOperator  Operator===  OutDataTypeStr=boolean  RndMeth=Simplest
  Equal3 : RelationalOperator  OutDataTypeStr=boolean  RndMeth=Simplest
  Equal4 : RelationalOperator  Operator===  OutDataTypeStr=boolean  RndMeth=Simplest
  Equal5 : RelationalOperator  Operator===  OutDataTypeStr=boolean  RndMeth=Simplest
  Logical Operator1 : Logic  Operator=NOT  AllPortsSameDT=off  OutDataTypeStr=boolean
  Logical Operator16 : Logic  Operator=NOT  AllPortsSameDT=off  OutDataTypeStr=boolean
  Logical Operator2 : Logic  Inputs=3  AllPortsSameDT=off  OutDataTypeStr=boolean
  Logical Operator3 : Logic  Inputs=3  AllPortsSameDT=off  OutDataTypeStr=boolean
  Logical Operator4 : Logic  AllPortsSameDT=off  OutDataTypeStr=boolean
  Logical Operator5 : Logic  Operator=OR  Inputs=4  AllPortsSameDT=off  OutDataTypeStr=boolean
  Logical Operator6 : Logic  Operator=NOT  AllPortsSameDT=off  OutDataTypeStr=boolean
  Logical Operator7 : Logic  AllPortsSameDT=off  OutDataTypeStr=boolean
  Relational Operator : RelationalOperator  Operator=>  OutDataTypeStr=boolean  RndMeth=Simplest
  Switch1 : Switch  Criteria=u2 ~= 0
  Switch2 : Switch  Criteria=u2 ~= 0
  Switch5 : Switch  Criteria=u2 ~= 0
  Terminator : Terminator
  Test Detection Criteria : hcu_lib/Basic_Blocks/Test Detection Criteria
  Timer1 : hcu_lib/Basic_Blocks/Timer
  Unit Delay3 : UnitDelay  SampleTime=-1  HasFrameUpgradeWarning=on
  VDDM_EPS1CSErrCFS_flg : Outport
  VDDM_EPS1CSErrDTC_raw32 : Outport  Port=2
  wires:
  Logical Operator4/1 -> Logical Operator5/3
  [VTQD_GearActualPosn_enum] -> Equal2/1
  Equal2/1 -> Logical Operator4/2
  Constant4/1 -> Equal2/2
  VTQD_GearActualPosn_enum/1 -> [VTQD_GearActualPosn_enum]
  [No_CAN1_BUS_OFF] -> Logical Operator3/1
  Logical Operator1/1 -> Logical Operator3/2
  [VDDM_EPS1NoComCFS_flg] -> Logical Operator1/1
  Equal1/1 -> Logical Operator3/3
  Constant1/1 -> Equal1/2
  [VPMM_PowerSta_enum] -> Equal1/1
  Logical Operator3/1 -> Switch1/2
  [VDDM_EPSCSErr_flg] -> Switch1/1
  Constant3/1 -> Switch1/3
  VPMM_PowerSta_enum/1 -> [VPMM_PowerSta_enum]
  DTC_clear_request/1 -> [DTC_clear_request]
  No_CAN1_BUS_OFF/1 -> [No_CAN1_BUS_OFF]
  VDDM_EPSCSErr_flg/1 -> [VDDM_EPSCSErr_flg]
  [VDDM_EPS1CSErrCFS_flg] -> VDDM_EPS1CSErrCFS_flg/1
  Logical Operator6/1 -> Timer1/1
  Constant2/1 -> Switch2/3
  [VDDM_EPSCSErr_flg] -> Switch2/1
  Timer1/1 -> Equal3/1
  Logical Operator2/1 -> Switch2/2
  Test Detection Criteria/1 -> [VDDM_EPS1CSErrDet_flg]  "VDDM_EPS1CSErrDet_flg"
  [task_time_s] -> Test Detection Criteria/2
  Constant41/1 -> Test Detection Criteria/4
  [VPMM_PowerSta_enum] -> Equal/1
  Switch1/1 -> Logical Operator6/1, Timer1/2
  Constant/1 -> Equal/2
  Switch2/1 -> Switch5/3
  Equal/1 -> Logical Operator2/3
  Constant6/1 -> Equal3/2
  Constant40/1 -> Test Detection Criteria/3
  task_time_s/1 -> [task_time_s]  "task_time_s"
  Constant9/1 -> Timer1/4
  [VDDM_EPS1NoComCFS_flg] -> Logical Operator16/1
  Logical Operator16/1 -> Logical Operator2/2
  [No_CAN1_BUS_OFF] -> Logical Operator2/1
  VDDM_EPS1NoComCFS_flg/1 -> [VDDM_EPS1NoComCFS_flg]
  [task_time_s] -> Timer1/3
  [VDDM_EPS1CSErrCFSRls_flg] -> Switch5/2
  Constant10/1 -> Switch5/1
  Switch5/1 -> Test Detection Criteria/1
  [VDDM_EPS1CSErrDet_flg] -> DTC_Info/1
  [VDDM_EPS1CSErrPass_flg] -> DTC_Info/2
  [VDDM_EPS1CSErrCFS_flg] -> DTC_Info/3
  [DTC_clear_request] -> DTC_Info/4
  DTC_Info/1 -> VDDM_EPS1CSErrDTC_raw32/1  "VDDM_EPS1CSErrDTC_raw32"
  Equal3/1 -> [VDDM_EPS1CSErrPass_flg]  "VDDM_EPS1CSErrPass_flg"
  DTC_Couter2/1 -> [VDDM_EPS1CSErrCFS_flg]  "VDDM_EPS1CSErrCFS_flg"
  [VDDM_EPS1CSErrDet_flg] -> DTC_Couter2/1
  [VDDM_EPS1CSErrCFSRls_flg] -> DTC_Couter2/2
  [VDDM_EPS1CSErrPass_flg] -> Logical Operator4/1
  Constant12/1 -> DTC_Couter2/3
  Constant11/1 -> Relational Operator/2
  Constant49/1 -> Equal4/2
  Equal5/1 -> Logical Operator7/2
  DTC_Couter2/2 -> Relational Operator/1  "VDDM_EPS1CSErrDTC_cnt"
  Constant52/1 -> Equal5/2
  Unit Delay3/1 -> Equal4/1
  Logical Operator7/1 -> Logical Operator5/1
  Equal4/1 -> Logical Operator7/1
  [DTC_clear_request] -> Logical Operator5/2
  [VPMM_PowerSta_enum] -> Equal5/1
  Constant13/1 -> Logical Operator5/4
  Logical Operator5/1 -> [VDDM_EPS1CSErrCFSRls_flg]  "VDDM_EPS1CSErrCFSRls_flg"
  Relational Operator/1 -> Terminator/1  "VDDM_EPS1CSErrDFS_flg"
  [VPMM_PowerSta_enum] -> Unit Delay3/1

== system ddm/DDM/DDM/VMC_DDM/Enabled Subsystem/EPS1 Lost Comm ==
  note: Release Condiction After Decision
  note: Diagnostics and Fault Handling
  note: Test Pass Criteria
  note: Test Detection Criteria
  task_time_s : Inport
  VPMM_PowerSta_enum : Inport  Port=2
  VDDM_EPS1NoCom_flg : Inport  Port=3
  No_CAN1_BUS_OFF : Inport  Port=4
  DTC_clear_request : Inport  Port=5
  VTQD_GearActualPosn_enum : Inport  Port=6
  Constant1 : Constant  Value=ZERO_INT
  Constant16 : Constant  Value=TRUE
  Constant18 : Constant  Value=KDDM_EPS1NoComPassTO_s
  Constant19 : Constant  Value=KDDM_EPS1NoComPassTO_s
  Constant2 : Constant  Value=FALSE
  Constant26 : Constant  Value=ENUM_PWRSTASW_OFF
  Constant27 : Constant  Value=FALSE
  Constant28 : Constant  Value=ENUM_PWRSTASW_OFF
  Constant3 : Constant  Value=KDDM_EPS1NoComDTC_cnt
  Constant4 : Constant  Value=ENUM_GEARACTUALPOSN_P
  Constant40 : Constant  Value=KDDM_EPS1NoComDTC_cnt
  Constant41 : Constant  Value=KDDM_EPS1NoComDetTO_s
  Constant49 : Constant  Value=ENUM_POWERSTA_OFF
  Constant52 : Constant  Value=ENUM_POWERSTA_STANDBY
  Constant8 : Constant  Value=KDDM_VMCDiagnosisOffSW_flg
  DTC_Couter2 : hcu_lib/Basic_Blocks/DTC_Couter
  DTC_Info : hcu_lib/Basic_Blocks/DTC_Info
  Equal : RelationalOperator  Operator=~=  OutDataTypeStr=boolean  RndMeth=Simplest
  Equal1 : RelationalOperator  Operator===  OutDataTypeStr=boolean  RndMeth=Simplest
  Equal2 : RelationalOperator  Operator=~=  OutDataTypeStr=boolean  RndMeth=Simplest
  Equal3 : RelationalOperator  OutDataTypeStr=boolean  RndMeth=Simplest
  Equal4 : RelationalOperator  Operator===  OutDataTypeStr=boolean  RndMeth=Simplest
  Equal8 : RelationalOperator  Operator===  OutDataTypeStr=boolean  RndMeth=Simplest
  Logical Operator{1..2,5,11} (4 alike) : Logic  AllPortsSameDT=off  OutDataTypeStr=boolean
  Logical Operator10 : Logic  Operator=OR  Inputs=4  AllPortsSameDT=off  OutDataTypeStr=boolean
  Logical Operator6 : Logic  Operator=NOT  AllPortsSameDT=off  OutDataTypeStr=boolean
  Relational Operator : RelationalOperator  Operator=>  OutDataTypeStr=boolean  RndMeth=Simplest
  Switch1 : Switch  Criteria=u2 ~= 0
  Switch5 : Switch  Criteria=u2 ~= 0
  Switch6 : Switch  Criteria=u2 ~= 0
  Terminator : Terminator
  Test Detection Criteria : hcu_lib/Basic_Blocks/Test Detection Criteria
  Timer1 : hcu_lib/Basic_Blocks/Timer
  Unit Delay3 : UnitDelay  SampleTime=-1  HasFrameUpgradeWarning=on
  VDDM_EPS1NoComCFS_flg : Outport
  VDDM_EPS1NoComDTC_raw32 : Outport  Port=2
  wires:
  Equal4/1 -> Logical Operator1/2
  Logical Operator1/1 -> Logical Operator10/3
  Constant4/1 -> Equal4/2
  [VTQD_GearActualPosn_enum] -> Equal4/1
  VTQD_GearActualPosn_enum/1 -> [VTQD_GearActualPosn_enum]
  [VDDM_EPS1NoComCFS_flg] -> VDDM_EPS1NoComCFS_flg/1
  Constant3/1 -> DTC_Couter2/3
  Constant1/1 -> Relational Operator/2
  Logical Operator11/1 -> Logical Operator10/1
  DTC_Couter2/1 -> [VDDM_EPS1NoComCFS_flg]  "VDDM_EPS1NoComCFS_flg"
  Logical Operator10/1 -> [VDDM_EPS1NoComCFSRls_flg]  "VDDM_EPS1NoComCFSRls_flg"
  [VDDM_EPS1NoComCFSRls_flg] -> DTC_Couter2/2
  [VPMM_PowerSta_enum] -> Equal8/1
  [VPMM_PowerSta_enum] -> Unit Delay3/1
  Equal1/1 -> Logical Operator11/1
  Constant49/1 -> Equal1/2
  [VDDM_EPS1NoComDet_flg] -> DTC_Couter2/1
  Relational Operator/1 -> Terminator/1  "VDDM_EPS1NoComDFS_flg"
  [VDDM_EPS1NoComPass_flg] -> Logical Operator1/1
  Equal8/1 -> Logical Operator11/2
  Constant52/1 -> Equal8/2
  DTC_Couter2/2 -> Relational Operator/1  "VDDM_EPS1NoComDTC_cnt"
  Unit Delay3/1 -> Equal1/1
  [DTC_clear_request] -> Logical Operator10/2
  Constant8/1 -> Logical Operator10/4
  Equal3/1 -> [VDDM_EPS1NoComPass_flg]  "VDDM_EPS1NoComPass_flg"
  Constant2/1 -> Switch1/1
  Switch5/1 -> Switch1/3
  Switch1/1 -> Test Detection Criteria/1
  [VDDM_EPS1NoComCFSRls_flg] -> Switch1/2
  [DTC_clear_request] -> DTC_Info/4
  Constant41/1 -> Test Detection Criteria/4
  [VDDM_EPS1NoComPass_flg] -> DTC_Info/2
  [VDDM_EPS1NoComDet_flg] -> DTC_Info/1
  [VDDM_EPS1NoComCFS_flg] -> DTC_Info/3
  DTC_Info/1 -> VDDM_EPS1NoComDTC_raw32/1  "VDDM_EPS1NoComDTC_raw32"
  [task_time_s] -> Timer1/3
  [VPMM_PowerSta_enum] -> Equal2/1
  [VPMM_PowerSta_enum] -> Equal/1
  Constant18/1 -> Timer1/4
  Switch6/1 -> Timer1/2, Logical Operator6/1
  Constant28/1 -> Equal2/2
  [VDDM_EPS1NoCom_flg] -> Switch5/1
  [VDDM_EPS1NoCom_flg] -> Switch6/1
  Equal2/1 -> Logical Operator5/2
  Constant40/1 -> Test Detection Criteria/3
  [No_CAN1_BUS_OFF] -> Logical Operator5/1
  Logical Operator5/1 -> Switch6/2
  Logical Operator2/1 -> Switch5/2
  Constant26/1 -> Equal/2
  [No_CAN1_BUS_OFF] -> Logical Operator2/1
  Constant27/1 -> Switch5/3
  Timer1/1 -> Equal3/1
  Equal/1 -> Logical Operator2/2
  [task_time_s] -> Test Detection Criteria/2
  Logical Operator6/1 -> Timer1/1
  Constant16/1 -> Switch6/3
  Constant19/1 -> Equal3/2
  No_CAN1_BUS_OFF/1 -> [No_CAN1_BUS_OFF]
  DTC_clear_request/1 -> [DTC_clear_request]
  task_time_s/1 -> [task_time_s]
  VDDM_EPS1NoCom_flg/1 -> [VDDM_EPS1NoCom_flg]
  VPMM_PowerSta_enum/1 -> [VPMM_PowerSta_enum]
  Test Detection Criteria/1 -> [VDDM_EPS1NoComDet_flg]  "VDDM_EPS1NoComDet_flg"

== system ddm/DDM/DDM/VMC_DDM/Enabled Subsystem/EPS1 Rolling Count Error  ==
  note: Test Pass Criteria
  note: Test Detection Criteria
  note: Release Condiction After Decision
  note: Diagnostics and Fault Handling
  task_time_s : Inport
  VDDM_EPSRCErr_flg : Inport  Port=2
  No_CAN1_BUS_OFF : Inport  Port=3
  VDDM_EPS1NoComCFS_flg : Inport  Port=4
  VPMM_PowerSta_enum : Inport  Port=5
  DTC_clear_request : Inport  Port=6
  VTQD_GearActualPosn_enum : Inport  Port=7
  Constant : Constant  Value=ENUM_POWERSTA_OFF
  Constant1 : Constant  Value=FALSE
  Constant16 : Constant  Value=ZERO_INT
  Constant2 : Constant  Value=FALSE
  Constant3 : Constant  Value=KDDM_EPS1RCErrDTC_cnt
  Constant4 : Constant  Value=ENUM_GEARACTUALPOSN_P
  Constant40 : Constant  Value=KDDM_EPS1RCErrDTC_cnt
  Constant41 : Constant  Value=KDDM_EPS1RCErrDetTO_s
  Constant49 : Constant  Value=ENUM_POWERSTA_OFF
  Constant5 : Constant  Value=ENUM_POWERSTA_OFF
  Constant52 : Constant  Value=ENUM_POWERSTA_STANDBY
  Constant6 : Constant  Value=KDDM_EPS1RCErrPassTO_s
  Constant7 : Constant  Value=TRUE
  Constant8 : Constant  Value=KDDM_VMCDiagnosisOffSW_flg
  Constant9 : Constant  Value=KDDM_EPS1RCErrPassTO_s
  DTC_Couter2 : hcu_lib/Basic_Blocks/DTC_Couter
  DTC_Info : hcu_lib/Basic_Blocks/DTC_Info
  Equal : RelationalOperator  Operator=~=  OutDataTypeStr=boolean  RndMeth=Simplest
  Equal1 : RelationalOperator  Operator===  OutDataTypeStr=boolean  RndMeth=Simplest
  Equal2 : RelationalOperator  Operator=~=  OutDataTypeStr=boolean  RndMeth=Simplest
  Equal3 : RelationalOperator  OutDataTypeStr=boolean  RndMeth=Simplest
  Equal4 : RelationalOperator  Operator===  OutDataTypeStr=boolean  RndMeth=Simplest
  Equal8 : RelationalOperator  Operator===  OutDataTypeStr=boolean  RndMeth=Simplest
  Logical Operator1 : Logic  AllPortsSameDT=off  OutDataTypeStr=boolean
  Logical Operator10 : Logic  Operator=OR  Inputs=4  AllPortsSameDT=off  OutDataTypeStr=boolean
  Logical Operator11 : Logic  AllPortsSameDT=off  OutDataTypeStr=boolean
  Logical Operator16 : Logic  Operator=NOT  AllPortsSameDT=off  OutDataTypeStr=boolean
  Logical Operator2 : Logic  Inputs=3  AllPortsSameDT=off  OutDataTypeStr=boolean
  Logical Operator4 : Logic  AllPortsSameDT=off  OutDataTypeStr=boolean
  Logical Operator6 : Logic  Operator=NOT  AllPortsSameDT=off  OutDataTypeStr=boolean
  Relational Operator : RelationalOperator  Operator=>  OutDataTypeStr=boolean  RndMeth=Simplest
  Switch2 : Switch  Criteria=u2 ~= 0
  Switch3 : Switch  Criteria=u2 ~= 0
  Switch5 : Switch  Criteria=u2 ~= 0
  Terminator : Terminator
  Test Detection Criteria : hcu_lib/Basic_Blocks/Test Detection Criteria
  Timer1 : hcu_lib/Basic_Blocks/Timer
  Unit Delay3 : UnitDelay  SampleTime=-1  HasFrameUpgradeWarning=on
  VDDM_EPS1RCErrCFS_flg : Outport
  VDDM_EPS1RCErrDTC_raw32 : Outport  Port=2
  wires:
  Logical Operator1/1 -> Logical Operator10/3
  [VDDM_EPS1RCErrPass_flg] -> Logical Operator1/1
  [VTQD_GearActualPosn_enum] -> Equal4/1
  Constant4/1 -> Equal4/2
  Equal4/1 -> Logical Operator1/2
  VTQD_GearActualPosn_enum/1 -> [VTQD_GearActualPosn_enum]
  VPMM_PowerSta_enum/1 -> [VPMM_PowerSta_enum]
  DTC_clear_request/1 -> [DTC_clear_request]
  No_CAN1_BUS_OFF/1 -> [No_CAN1_BUS_OFF]
  VDDM_EPSRCErr_flg/1 -> [VDDM_EPSRCErr_flg]
  [VDDM_EPS1RCErrCFS_flg] -> VDDM_EPS1RCErrCFS_flg/1
  Logical Operator6/1 -> Timer1/1
  Constant5/1 -> Equal2/2
  Constant2/1 -> Switch2/3
  Logical Operator4/1 -> Switch3/2
  Constant7/1 -> Switch3/3
  [VDDM_EPSRCErr_flg] -> Switch2/1
  Timer1/1 -> Equal3/1
  Logical Operator2/1 -> Switch2/2
  Test Detection Criteria/1 -> [VDDM_EPS1RCErrDet_flg]  "VDDM_EPS1RCErrDet_flg"
  [task_time_s] -> Test Detection Criteria/2
  Constant41/1 -> Test Detection Criteria/4
  [VPMM_PowerSta_enum] -> Equal/1
  Switch3/1 -> Logical Operator6/1, Timer1/2
  Constant/1 -> Equal/2
  Switch2/1 -> Switch5/3
  [VDDM_EPSRCErr_flg] -> Switch3/1
  [VPMM_PowerSta_enum] -> Equal2/1
  [No_CAN1_BUS_OFF] -> Logical Operator4/1
  Equal2/1 -> Logical Operator4/2
  Equal/1 -> Logical Operator2/3
  Equal3/1 -> [VDDM_EPS1RCErrPass_flg]  "VDDM_EPS1RCErrPass_flg"
  Constant6/1 -> Equal3/2
  Constant40/1 -> Test Detection Criteria/3
  task_time_s/1 -> [task_time_s]  "task_time_s"
  Constant9/1 -> Timer1/4
  [VDDM_EPS1NoComCFS_flg] -> Logical Operator16/1
  Logical Operator16/1 -> Logical Operator2/2
  [No_CAN1_BUS_OFF] -> Logical Operator2/1
  VDDM_EPS1NoComCFS_flg/1 -> [VDDM_EPS1NoComCFS_flg]
  [task_time_s] -> Timer1/3
  [VDDM_EPS1RCErrCFSRls_flg] -> Switch5/2
  Constant1/1 -> Switch5/1
  Switch5/1 -> Test Detection Criteria/1
  [VDDM_EPS1RCErrDet_flg] -> DTC_Info/1
  [VDDM_EPS1RCErrPass_flg] -> DTC_Info/2
  [VDDM_EPS1RCErrCFS_flg] -> DTC_Info/3
  [DTC_clear_request] -> DTC_Info/4
  DTC_Info/1 -> VDDM_EPS1RCErrDTC_raw32/1  "VDDM_EPS1RCErrDTC_raw32"
  DTC_Couter2/1 -> [VDDM_EPS1RCErrCFS_flg]  "VDDM_EPS1RCErrCFS_flg"
  [VPMM_PowerSta_enum] -> Unit Delay3/1
  [DTC_clear_request] -> Logical Operator10/2
  [VPMM_PowerSta_enum] -> Equal8/1
  Constant8/1 -> Logical Operator10/4
  Equal1/1 -> Logical Operator11/1
  Unit Delay3/1 -> Equal1/1
  Logical Operator11/1 -> Logical Operator10/1
  Constant49/1 -> Equal1/2
  DTC_Couter2/2 -> Relational Operator/1  "VDDM_EPS1RCErrDTC_cnt"
  Constant52/1 -> Equal8/2
  [VDDM_EPS1RCErrDet_flg] -> DTC_Couter2/1
  Logical Operator10/1 -> [VDDM_EPS1RCErrCFSRls_flg]  "VDDM_EPS1RCErrCFSRls_flg"
  [VDDM_EPS1RCErrCFSRls_flg] -> DTC_Couter2/2
  Constant16/1 -> Relational Operator/2
  Equal8/1 -> Logical Operator11/2
  Constant3/1 -> DTC_Couter2/3
  Relational Operator/1 -> Terminator/1  "VDDM_EPS1RCErrDFS_flg"

== system ddm/DDM/DDM/VMC_DDM/Enabled Subsystem/EPS1 Signal Error ==
  note: Release Condiction After Decision
  note: Diagnostics and Fault Handling
  note: Test Detection Criteria
  note: Test Pass Criteria
  task_time_s : Inport
  VINP_SASV_flg : Inport  Port=2
  No_CAN1_BUS_OFF : Inport  Port=3
  VDDM_EPS1NoComCFS_flg : Inport  Port=4
  VPMM_PowerSta_enum : Inport  Port=5
  DTC_clear_request : Inport  Port=6
  VDDM_EPS1RCErrCFS_flg : Inport  Port=7
  VDDM_EPS1CSErrCFS_flg : Inport  Port=8
  VTQD_GearActualPosn_enum : Inport  Port=9
  Constant : Constant  Value=ENUM_POWERSTA_OFF
  Constant1 : Constant  Value=ENUM_POWERSTA_OFF
  Constant10 : Constant  Value=FALSE
  Constant11 : Constant  Value=ZERO_INT
  Constant12 : Constant  Value=KDDM_EPSSigErrDTC_cnt
  Constant13 : Constant  Value=KDDM_VMCDiagnosisOffSW_flg
  Constant2 : Constant  Value=FALSE
  Constant3 : Constant  Value=TRUE
  Constant4 : Constant  Value=ENUM_GEARACTUALPOSN_P
  Constant40 : Constant  Value=KDDM_EPSSigErrDTC_cnt
  Constant41 : Constant  Value=KDDM_EPSSigErrDetTO_s
  Constant49 : Constant  Value=ENUM_POWERSTA_OFF
  Constant52 : Constant  Value=ENUM_POWERSTA_STANDBY
  Constant6 : Constant  Value=KDDM_EPSSigErrPassTO_s
  Constant9 : Constant  Value=KDDM_EPSSigErrPassTO_s
  DTC_Couter2 : hcu_lib/Basic_Blocks/DTC_Couter
  DTC_Info : hcu_lib/Basic_Blocks/DTC_Info
  Equal : RelationalOperator  Operator=~=  OutDataTypeStr=boolean  RndMeth=Simplest
  Equal1 : RelationalOperator  Operator=~=  OutDataTypeStr=boolean  RndMeth=Simplest
  Equal2 : RelationalOperator  Operator===  OutDataTypeStr=boolean  RndMeth=Simplest
  Equal3 : RelationalOperator  OutDataTypeStr=boolean  RndMeth=Simplest
  Equal4 : RelationalOperator  Operator===  OutDataTypeStr=boolean  RndMeth=Simplest
  Equal5 : RelationalOperator  Operator===  OutDataTypeStr=boolean  RndMeth=Simplest
  Logical Operator{1,4,6,8..12,16} (9 alike) : Logic  Operator=NOT  AllPortsSameDT=off  OutDataTypeStr=boolean
  Logical Operator13 : Logic  AllPortsSameDT=off  OutDataTypeStr=boolean
  Logical Operator2 : Logic  Inputs=5  AllPortsSameDT=off  OutDataTypeStr=boolean
  Logical Operator3 : Logic  Inputs=5  AllPortsSameDT=off  OutDataTypeStr=boolean
  Logical Operator5 : Logic  Operator=OR  Inputs=4  AllPortsSameDT=off  OutDataTypeStr=boolean
  Logical Operator7 : Logic  AllPortsSameDT=off  OutDataTypeStr=boolean
  Relational Operator : RelationalOperator  Operator=>  OutDataTypeStr=boolean  RndMeth=Simplest
  Switch1 : Switch  Criteria=u2 ~= 0
  Switch2 : Switch  Criteria=u2 ~= 0
  Switch5 : Switch  Criteria=u2 ~= 0
  Terminator : Terminator
  Test Detection Criteria : hcu_lib/Basic_Blocks/Test Detection Criteria
  Timer1 : hcu_lib/Basic_Blocks/Timer
  Unit Delay3 : UnitDelay  SampleTime=-1  HasFrameUpgradeWarning=on
  VDDM_EPSSigErrCFS_flg : Outport
  VDDM_EPSSigErrDTC_raw32 : Outport  Port=2
  wires:
  [VDDM_EPSSigErrPass_flg] -> Logical Operator13/1
  Logical Operator13/1 -> Logical Operator5/3
  Constant4/1 -> Equal2/2
  [VTQD_GearActualPosn_enum] -> Equal2/1
  Equal2/1 -> Logical Operator13/2
  VTQD_GearActualPosn_enum/1 -> [VTQD_GearActualPosn_enum]
  Logical Operator10/1 -> Switch1/1
  Constant1/1 -> Equal1/2
  Constant3/1 -> Switch1/3
  [VDDM_EPS1NoComCFS_flg] -> Logical Operator1/1
  [VPMM_PowerSta_enum] -> Equal1/1
  Logical Operator1/1 -> Logical Operator3/2
  [VDDM_EPS1RCErrCFS_flg] -> Logical Operator11/1
  Logical Operator11/1 -> Logical Operator3/3
  Equal1/1 -> Logical Operator3/5
  [VINP_SASV_flg] -> Logical Operator10/1
  [VDDM_EPS1CSErrCFS_flg] -> Logical Operator12/1
  Logical Operator12/1 -> Logical Operator3/4
  Logical Operator3/1 -> Switch1/2
  [No_CAN1_BUS_OFF] -> Logical Operator3/1
  [VDDM_EPS1CSErrCFS_flg] -> Logical Operator9/1
  Logical Operator9/1 -> Logical Operator2/4
  Logical Operator8/1 -> Logical Operator2/3
  [VDDM_EPS1RCErrCFS_flg] -> Logical Operator8/1
  Logical Operator4/1 -> Switch2/1
  VDDM_EPS1CSErrCFS_flg/1 -> [VDDM_EPS1CSErrCFS_flg]
  VDDM_EPS1RCErrCFS_flg/1 -> [VDDM_EPS1RCErrCFS_flg]
  [VPMM_PowerSta_enum] -> Unit Delay3/1
  Relational Operator/1 -> Terminator/1  "VDDM_EPSSigErrDFS_flg"
  Logical Operator5/1 -> [VDDM_EPSSigErrCFSRls_flg]  "VDDM_EPSSigErrCFSRls_flg"
  Constant13/1 -> Logical Operator5/4
  [VPMM_PowerSta_enum] -> Equal5/1
  [DTC_clear_request] -> Logical Operator5/2
  Equal4/1 -> Logical Operator7/1
  Logical Operator7/1 -> Logical Operator5/1
  Unit Delay3/1 -> Equal4/1
  Constant52/1 -> Equal5/2
  DTC_Couter2/2 -> Relational Operator/1  "VDDM_EPSSigErrDTC_cnt"
  Equal5/1 -> Logical Operator7/2
  Constant49/1 -> Equal4/2
  Constant11/1 -> Relational Operator/2
  Constant12/1 -> DTC_Couter2/3
  [VDDM_EPSSigErrCFSRls_flg] -> DTC_Couter2/2
  [VDDM_EPSSigErrDet_flg] -> DTC_Couter2/1
  DTC_Couter2/1 -> [VDDM_EPSSigErrCFS_flg]  "VDDM_EPSSigErrCFS_flg"
  Equal3/1 -> [VDDM_EPSSigErrPass_flg]  "VDDM_EPSSigErrPass_flg"
  DTC_Info/1 -> VDDM_EPSSigErrDTC_raw32/1  "VDDM_EPSSigErrDTC_raw32"
  [DTC_clear_request] -> DTC_Info/4
  [VDDM_EPSSigErrCFS_flg] -> DTC_Info/3
  [VDDM_EPSSigErrPass_flg] -> DTC_Info/2
  [VDDM_EPSSigErrDet_flg] -> DTC_Info/1
  Switch5/1 -> Test Detection Criteria/1
  Constant10/1 -> Switch5/1
  [VDDM_EPSSigErrCFSRls_flg] -> Switch5/2
  [task_time_s] -> Timer1/3
  VDDM_EPS1NoComCFS_flg/1 -> [VDDM_EPS1NoComCFS_flg]
  [No_CAN1_BUS_OFF] -> Logical Operator2/1
  Logical Operator16/1 -> Logical Operator2/2
  [VDDM_EPS1NoComCFS_flg] -> Logical Operator16/1
  Constant9/1 -> Timer1/4
  task_time_s/1 -> [task_time_s]  "task_time_s"
  Constant40/1 -> Test Detection Criteria/3
  Constant6/1 -> Equal3/2
  Equal/1 -> Logical Operator2/5
  Switch2/1 -> Switch5/3
  Constant/1 -> Equal/2
  Switch1/1 -> Timer1/2, Logical Operator6/1
  [VPMM_PowerSta_enum] -> Equal/1
  Constant41/1 -> Test Detection Criteria/4
  [task_time_s] -> Test Detection Criteria/2
  Test Detection Criteria/1 -> [VDDM_EPSSigErrDet_flg]  "VDDM_EPSSigErrDet_flg"
  Logical Operator2/1 -> Switch2/2
  Timer1/1 -> Equal3/1
  [VINP_SASV_flg] -> Logical Operator4/1
  Constant2/1 -> Switch2/3
  Logical Operator6/1 -> Timer1/1
  [VDDM_EPSSigErrCFS_flg] -> VDDM_EPSSigErrCFS_flg/1
  VINP_SASV_flg/1 -> [VINP_SASV_flg]
  No_CAN1_BUS_OFF/1 -> [No_CAN1_BUS_OFF]
  DTC_clear_request/1 -> [DTC_clear_request]
  VPMM_PowerSta_enum/1 -> [VPMM_PowerSta_enum]
